simulink model "tank"  (R2017a)
settings: Solver=VariableStepAuto  StartTime=0.0  StopTime=100  RelTol=1e-3
values from neighbouring files (symbols this model uses):
  h1 = 0    [TankValues.m]
  h2 = 0    [TankValues.m]
  inflow1 = 0.2    [TankValues.m]
settings Model: Creator=kejo5874  LastModifiedBy=kejo5874

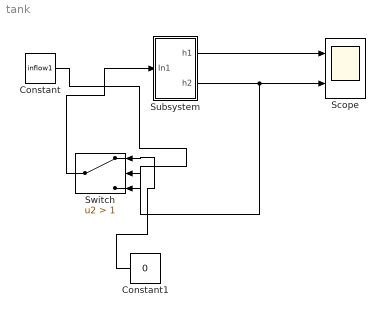
== system tank ==
  Constant : Constant  Value=inflow1
  Constant1 : Constant  Value=0
  Scope : Scope  NumInputPorts=2
  Subsystem : Subsystem
  Switch : Switch  Criteria=u2 > Threshold  Threshold=1
  wires:
  Subsystem/1(h1) -> Scope/1
  Subsystem/2(h2) -> Switch/2, Scope/2
  Constant/1 -> Switch/3
  Switch/1 -> Subsystem/1(In1)
  Constant1/1 -> Switch/1

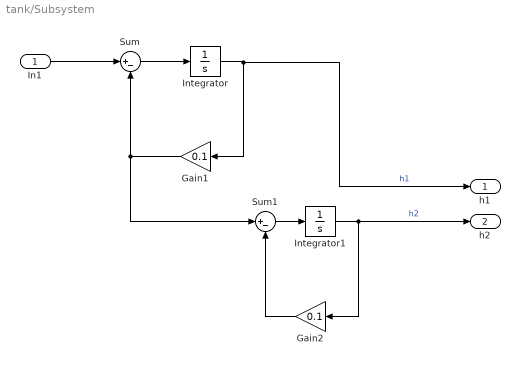
== system tank/Subsystem ==
  In1 : Inport
  Gain1 : Gain  Gain=0.1
  Gain2 : Gain  Gain=0.1
  Integrator : Integrator  InitialCondition=h1
  Integrator1 : Integrator  InitialCondition=h2
  Sum : Sum  Inputs=|+-
  Sum1 : Sum  Inputs=|+-
  h1 : Outport
  h2 : Outport  Port=2
  wires:
  Integrator1/1 -> h2/1, Gain2/1  "h2"
  Sum1/1 -> Integrator1/1
  Gain2/1 -> Sum1/2
  Sum/1 -> Integrator/1
  Integrator/1 -> h1/1, Gain1/1  "h1"
  Gain1/1 -> Sum1/1, Sum/2
  In1/1 -> Sum/1
